simulink model "RadarSimulinkProjectRev004"  (R2024a)
settings: Solver=VariableStepAuto  StartTime=0.0  StopTime=0.012  RelTol=1e-3
values from neighbouring files (symbols this model uses):
  AngleTime = SweepTime/10    (= 10000)    [InitializationOfVariablesRev000.m]    (also in InitializationOfVariablesRev001.m; InitializationOfVariablesRev002.m = 2000; InitializationOfVariablesRev003.m = 20000; InitializationOfVariablesRev004.m = 2097152)
  ASR_LUT = Rsamp    [InitializationOfVariablesRev003.m]    (also in InitializationOfVariablesRev004.m = round((R*2*SystemFs)/c); InitializationOfVariablesRev005.m = round((R*2*SystemFs)/c))
  Btn_Debounce = 20000    [InitializationOfVariablesRev003.m]    (also in InitializationOfVariablesRev004.m; InitializationOfVariablesRev005.m)
  ChirpNc = 128    [InitializationOfVariablesRev004.m]    (also in InitializationOfVariablesRev005.m)
  ChirpSizeLength = length(FCW)    [InitializationOfVariablesRev004.m]    (also in InitializationOfVariablesRev005.m = 16384)
  FreqDeltaPeriod = 54    [InitializationOfVariablesRev003.m]    (also in InitializationOfVariablesRev004.m = 1)
  RXFFTLength = 4096    [InitializationOfVariablesRev003.m]    (also in InitializationOfVariablesRev004.m = 1024; InitializationOfVariablesRev005.m = 2048)
  SweepTime = 100000    [InitializationOfVariablesRev000.m]    (also in InitializationOfVariablesRev001.m; InitializationOfVariablesRev002.m = 20000; InitializationOfVariablesRev003.m = 200000; InitializationOfVariablesRev004.m = 23068672)
undefined symbols (not defined in the file or in its folder): SignalGenerationForAnalysis, Subsystem, xc7a200tfbg676
libraries: hdlBasic x323, hdlDSPIP x12, hdlUtilities x11, vmcUtilities x1
(part 3 of 3)

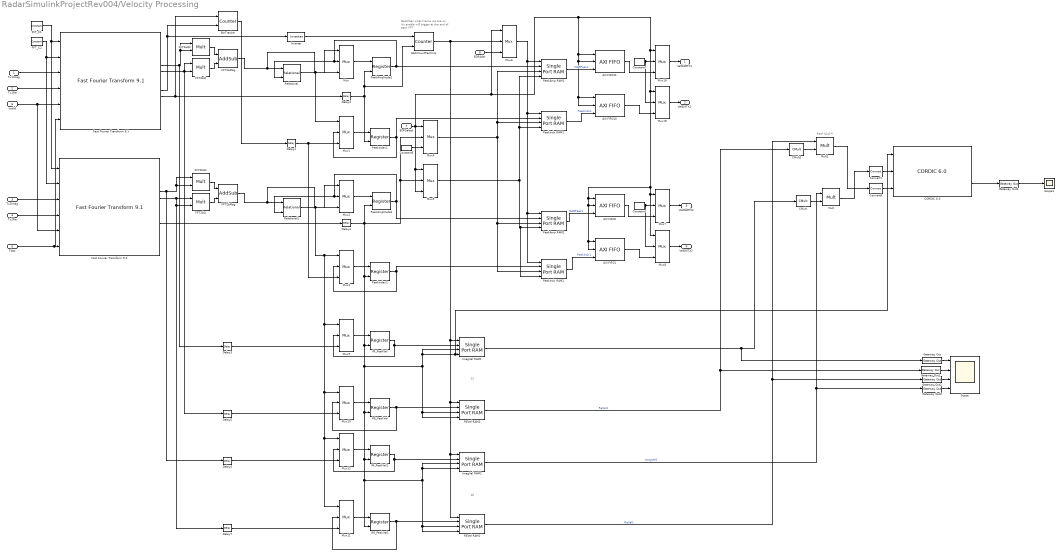
== system RadarSimulinkProjectRev004/Velocity Processing ==
  note: Real (z2z1*)
  note: Z1
  note: Describes what Frame we are on, it's enable will trigger at the end of each FFT
  note: Z2
  Tx1Imag : Inport
  Tx1Re : Inport  Port=2
  Tx2Imag : Inport  Port=3
  Tx2Re : Inport  Port=4
  Tlast : Inport  Port=5
  tvalid : Inport  Port=6
  EOFSelect : Inport  Port=7
  EOFAddr : Inport  Port=8
  AXI FIFO{1..2,10..11} (4 alike) : hdlBasic/AXI FIFO  input_depth_axis=1K  actual_fifo_depth_label=1026  enable_tdata=on  enable_tdest=off  enable_tstrb=off  enable_tready=on  enable_tid=off  enable_tuser=off  enable_tkeep=off  enable_tlast=off  has_aresetn=off  enable_data_counts_axis=off  fifo_implementation_type_axis=Common Clock Block RAM  trim_axipin_name=on  programmable_full_type_axis=Full  full_threshold_assert_value_axis=0  programmable_empty_type_axis=Empty  empty_threshold_assert_value_axis=1022  underflow_flag_axi=0  underflow_sense_axi=Active High  overflow_flag_axi=0  overflow_sense_axi=Active High  simulation_type=fast_sim  XmcBlockStatus=1  maskContainerNames=tabcontainer1  block_type=axi_fifo  block_config=sysgen:AXI_FIFO_config
  AddrCountPerChirp : hdlBasic/Counter  cnt_type=Count limited  cnt_to=10  operation=Up  start_count=0  cnt_by_val=1  arith_type=Unsigned  n_bits=7  bin_pt=0  load_pin=off  rst=on  en=on  explicit_period=Explicit  period=1/200e6  use_behavioral_HDL=off  implementation=Fabric  XmcBlockStatus=1  maskContainerNames=group1  block_type=counter  block_config=sysgen:Counter_config  block_width=531  block_height=1023
  BinTracker : hdlBasic/Counter  cnt_type=Count limited  cnt_to=ChirpNc-1  operation=Up  start_count=0  cnt_by_val=1  arith_type=Unsigned  n_bits=14  bin_pt=0  load_pin=off  rst=on  en=on  explicit_period=Explicit  period=1/200e6  use_behavioral_HDL=off  implementation=Fabric  XmcBlockStatus=1  maskContainerNames=group1  block_type=counter  block_config=sysgen:Counter_config  block_width=531  block_height=1023
  CMult : hdlBasic/CMult  const=-1  gui_display_data_type=Fixed-point  const_n_bits=16  const_bin_pt=14  float_type=Single  exp_bits=8  fraction_bits=24  en=off  latency=0  precision=Full  arith_type="Signed  (2's comp)"  n_bits=16  bin_pt=14  quantization=Truncate  overflow=Wrap  use_behavioral_HDL=off  mem_type=Distributed RAM  pipeline=off  XmcBlockStatus=1  maskContainerNames=tabcontainer1  block_type=cmult  block_config=sysgen:CMult_config
      settings: infoedit=[]
  CMult1 : hdlBasic/CMult  const=-1  gui_display_data_type=Fixed-point  const_n_bits=16  const_bin_pt=14  float_type=Single  exp_bits=8  fraction_bits=24  en=off  latency=0  precision=Full  arith_type="Signed  (2's comp)"  n_bits=16  bin_pt=14  quantization=Truncate  overflow=Wrap  use_behavioral_HDL=off  mem_type=Distributed RAM  pipeline=off  XmcBlockStatus=1  maskContainerNames=tabcontainer1  block_type=cmult  block_config=sysgen:CMult_config
      settings: infoedit=[]
  CORDIC 6.0 : hdlDSPIP/CORDIC 6.0   functional_selection=Arc_Tan  architectural_configuration=Parallel  pipelining_mode=Maximum  data_format=SignedFraction  phase_format=Radians  input_width=16  output_width=16  round_mode=Truncate  iterations=0  precision=0  compensation_scaling=No_Scale_Compensation  coarse_rotation=on  aclken=off  aresetn=off  out_tready=off  cartesian_has_tuser=off  cartesian_has_tlast=off  cartesian_tuser_width=1  phase_has_tuser=off  phase_has_tlast=off  phase_tuser_width=1  out_tlast_behv=Null  flow_control=NonBlocking  optimize_goal=Resources  trim_axipin_name=on  simulation_type=hybrid_sim  simulation_model=sysgen:cordic_v6_0  data_path_portlist={'s_axis_cartesian_tdata_imag', 's_axis_cartesian_tdata_real', 's_axis_phase_tdata_phase', 'm_axis_dout_tdata_imag', 'm_axis_dout_tdata_real', 'm_axis_dout_tdata_phase','m_axis_dout_tdata'}  ip_name=CORDIC  ip_version=6.0  dsptool_ready=true  ipcore_usecache=true  ipcore_useipmodelcache=true  wrapper_available=true  port_translation_map={ 'aclken' => 'en', 'aresetn' => 'rst' }  XmcBlockStatus=1  maskContainerNames=group15  block_type=cordic_v6_0  block_config=sysgen:rodinimport_config  block_width=800
  Constant1 : hdlBasic/Constant  const=0  gui_display_data_type=Fixed-point  arith_type=Signed (2's comp)  n_bits=16  bin_pt=15  preci_type=Single  exp_width=8  frac_width=24  explicit_period=on  period=1/200e6  XmcBlockStatus=1  maskContainerNames=tabcontainer1  block_type=constant  block_config=sysgen:Constant_config
  Constant5 : hdlBasic/Constant  const=0  gui_display_data_type=Boolean  arith_type=Boolean  n_bits=16  bin_pt=15  preci_type=Single  exp_width=8  frac_width=24  explicit_period=on  period=1/200e6  XmcBlockStatus=1  maskContainerNames=tabcontainer1  block_type=constant  block_config=sysgen:Constant_config
  Constant7 : hdlBasic/Constant  const=0  gui_display_data_type=Fixed-point  arith_type=Signed (2's comp)  n_bits=16  bin_pt=15  preci_type=Single  exp_width=8  frac_width=24  explicit_period=on  period=1/200e6  XmcBlockStatus=1  maskContainerNames=tabcontainer1  block_type=constant  block_config=sysgen:Constant_config
  Convert7 : hdlBasic/Convert  gui_display_data_type=Fixed-point  arith_type=Signed (2's comp)  n_bits=33  bin_pt=31  float_type=Single  exp_bits=8  fraction_bits=24  quantization=Truncate  overflow=Wrap  en=off  latency=0  pipeline=off  XmcBlockStatus=1  maskContainerNames=group2  block_type=convert  block_config=sysgen:Convert_config  block_width=595  block_height=885
  Convert8 : hdlBasic/Convert  gui_display_data_type=Fixed-point  arith_type=Signed (2's comp)  n_bits=33  bin_pt=31  float_type=Single  exp_bits=8  fraction_bits=24  quantization=Truncate  overflow=Wrap  en=off  latency=0  pipeline=off  XmcBlockStatus=1  maskContainerNames=group2  block_type=convert  block_config=sysgen:Convert_config  block_width=595  block_height=885
  Delay{1,3,5..7} (5 alike) : hdlBasic/Delay  rst=off  en=off  latency=3  reg_retiming=off  XmcBlockStatus=1  maskContainerNames=group1  block_type=delay  block_config=sysgen:Delay_config
  Delay2 : hdlBasic/Delay  rst=off  en=off  latency=1  reg_retiming=off  XmcBlockStatus=1  maskContainerNames=group1  block_type=delay  block_config=sysgen:Delay_config
  Delay4 : hdlBasic/Delay  rst=off  en=off  latency=1  reg_retiming=off  XmcBlockStatus=1  maskContainerNames=group1  block_type=delay  block_config=sysgen:Delay_config
  FFT2aI2 : hdlBasic/Mult  precision=Full  arith_type="Signed  (2's comp)"  n_bits=16  bin_pt=14  quantization=Truncate  overflow=Wrap  en=off  latency=3  opt_float=off  fp_mult_usage=No Usage  use_behavioral_HDL=off  opt=Speed  use_embedded=on  optimum_pipeline=off  pipeline=on  use_rpm=on  placement_style=Triangular  XmcBlockStatus=1  maskContainerNames=group1  block_type=mult  block_config=sysgen:Mult_config  block_width=598  block_height=876
  FFT2aMag : hdlBasic/AddSub  mode=Addition  use_carryin=off  use_carryout=off  en=off  latency=0  precision=Full  arith_type=Unsigned  n_bits=16  bin_pt=14  quantization=Truncate  overflow=Wrap  use_behavioral_HDL=off  hw_selection=Fabric  pipelined=off  XmcBlockStatus=1  maskContainerNames=tabcontainer1  block_type=addsub  block_config=sysgen:Addsub_config
  FFT2aQ2 : hdlBasic/Mult  precision=Full  arith_type="Signed  (2's comp)"  n_bits=16  bin_pt=14  quantization=Truncate  overflow=Wrap  en=off  latency=3  opt_float=off  fp_mult_usage=No Usage  use_behavioral_HDL=off  opt=Speed  use_embedded=on  optimum_pipeline=off  pipeline=on  use_rpm=on  placement_style=Triangular  XmcBlockStatus=1  maskContainerNames=group1  block_type=mult  block_config=sysgen:Mult_config  block_width=598  block_height=876
  FFT2bI2 : hdlBasic/Mult  precision=Full  arith_type="Signed  (2's comp)"  n_bits=16  bin_pt=14  quantization=Truncate  overflow=Wrap  en=off  latency=3  opt_float=off  fp_mult_usage=No Usage  use_behavioral_HDL=off  opt=Speed  use_embedded=on  optimum_pipeline=off  pipeline=on  use_rpm=on  placement_style=Triangular  XmcBlockStatus=1  maskContainerNames=group1  block_type=mult  block_config=sysgen:Mult_config  block_width=598  block_height=876
  FFT2bMag : hdlBasic/AddSub  mode=Addition  use_carryin=off  use_carryout=off  en=off  latency=0  precision=Full  arith_type=Unsigned  n_bits=16  bin_pt=14  quantization=Truncate  overflow=Wrap  use_behavioral_HDL=off  hw_selection=Fabric  pipelined=off  XmcBlockStatus=1  maskContainerNames=tabcontainer1  block_type=addsub  block_config=sysgen:Addsub_config
  FFT2bQ2 : hdlBasic/Mult  precision=Full  arith_type="Signed  (2's comp)"  n_bits=16  bin_pt=14  quantization=Truncate  overflow=Wrap  en=off  latency=3  opt_float=off  fp_mult_usage=No Usage  use_behavioral_HDL=off  opt=Speed  use_embedded=on  optimum_pipeline=off  pipeline=on  use_rpm=on  placement_style=Triangular  XmcBlockStatus=1  maskContainerNames=group1  block_type=mult  block_config=sysgen:Mult_config  block_width=598  block_height=876
  FFT_C1 : hdlBasic/Constant  const=1.0  gui_display_data_type=Fixed-point  arith_type=Unsigned  n_bits=1  bin_pt=0  preci_type=Single  exp_width=8  frac_width=24  explicit_period=on  period=1/200e6  XmcBlockStatus=1  maskContainerNames=tabcontainer1  block_type=constant  block_config=sysgen:Constant_config
  FFT_C2 : hdlBasic/Constant  const=1.0  gui_display_data_type=Boolean  arith_type=Boolean  n_bits=1  bin_pt=0  preci_type=Single  exp_width=8  frac_width=24  explicit_period=on  period=1/200e6  XmcBlockStatus=1  maskContainerNames=tabcontainer1  block_type=constant  block_config=sysgen:Constant_config
  Fast Fourier Transform 9.1 : hdlDSPIP/Fast Fourier Transform 9.1   transform_length=128  target_clock_frequency=250  target_data_throughput=50  implementation_options=pipelined_streaming_io  run_time_configurable_transform_length=off  enable_ssr=off  super_sample_rates=1  data_format=fixed_point  phase_factor_width=24  scaling_options=block_floating_point  rounding_modes=truncation  aclken=off  aresetn=off  output_ordering=natural_order  cyclic_prefix_insertion=off  throttle_scheme=realtime  xk_index=on  ovflo=off  trim_axipin_name=on  memory_options_data=block_ram  memory_options_phase_factors=block_ram  number_of_stages_using_block_ram_for_data_and_phase_factors=2  memory_options_reorder=block_ram  memory_options_hybrid=off  complex_mult_type=use_mults_resources  butterfly_type=use_xtremedsp_slices  simulation_type=hybrid_sim  simulation_model=sysgen:xfftv9_cmodel  data_path_portlist={ 's_axis_data_tdata', 'm_axis_data_tdata', 'm_axis_status_tdata', 'event_fft_overflow' }  channels=1  input_ordering=natural_order  input_width=16  ip_name=Fast Fourier Transform  ip_version=9.1  dsptool_ready=true  ipcore_usecache=true  ipcore_useipmodelcache=true  wrapper_available=true  port_translation_map={ 'aclken' => 'en', 'aresetn' => 'rst'}  XmcBlockStatus=1  maskContainerNames=tabcontainer1  block_type=xfft_v9_1  block_config=sysgen:rodinimport_config
  Fast Fourier Transform 9.2 : hdlDSPIP/Fast Fourier Transform 9.1   transform_length=128  target_clock_frequency=250  target_data_throughput=50  implementation_options=pipelined_streaming_io  run_time_configurable_transform_length=off  enable_ssr=off  super_sample_rates=1  data_format=fixed_point  phase_factor_width=24  scaling_options=block_floating_point  rounding_modes=truncation  aclken=off  aresetn=off  output_ordering=natural_order  cyclic_prefix_insertion=off  throttle_scheme=realtime  xk_index=on  ovflo=off  trim_axipin_name=on  memory_options_data=block_ram  memory_options_phase_factors=block_ram  number_of_stages_using_block_ram_for_data_and_phase_factors=2  memory_options_reorder=block_ram  memory_options_hybrid=off  complex_mult_type=use_mults_resources  butterfly_type=use_xtremedsp_slices  simulation_type=hybrid_sim  simulation_model=sysgen:xfftv9_cmodel  data_path_portlist={ 's_axis_data_tdata', 'm_axis_data_tdata', 'm_axis_status_tdata', 'event_fft_overflow' }  channels=1  input_ordering=natural_order  input_width=16  ip_name=Fast Fourier Transform  ip_version=9.1  dsptool_ready=true  ipcore_usecache=true  ipcore_useipmodelcache=true  wrapper_available=true  port_translation_map={ 'aclken' => 'en', 'aresetn' => 'rst'}  XmcBlockStatus=1  maskContainerNames=tabcontainer1  block_type=xfft_v9_1  block_config=sysgen:rodinimport_config
  Gateway Out{,1..4} (5 alike) : hdlBasic/Gateway Out  inherit_from_input=off  bool_to_boolean=off  hdl_port=on  rows=1  columns=1  UseAsDAC=off  DACChannel='1'  interface=None  automatic_assignment=on  address_offset=hex2dec('00')  intf_name=''  intf_description=''  timing_constraint=None  locs_specified=off  LOCs={}  io_standard={}  XmcBlockStatus=1  maskContainerNames=group4  block_type=gatewayout  block_config=sysgen:gateway_out_config  block_width_w=590  block_height_w=620  block_width=620  block_height=750
  IM_PeakVal : hdlBasic/Register  init=0  rst=on  en=off  XmcBlockStatus=1  maskContainerNames=tabcontainer1  block_type=register  block_config=sysgen:Register_config
  IM_PeakVal1 : hdlBasic/Register  init=0  rst=on  en=off  XmcBlockStatus=1  maskContainerNames=tabcontainer1  block_type=register  block_config=sysgen:Register_config
  ImagVal RAM1 : hdlBasic/Single Port RAM  depth=ChirpNc  initVector=0  distributed_mem=Block RAM  write_mode=Read After Write  rst=off  init_reg=0  en=on  optimize_latency=off  latency=1  optimize=Area  dbl_ovrd=off  simulation_type=fast_sim  XmcBlockStatus=1  maskContainerNames=tabcontainer1  block_type=spram  block_config=sysgen:SPRAM_config
  ImagVal RAM2 : hdlBasic/Single Port RAM  depth=ChirpNc  initVector=0  distributed_mem=Block RAM  write_mode=Read After Write  rst=off  init_reg=0  en=on  optimize_latency=off  latency=1  optimize=Area  dbl_ovrd=off  simulation_type=fast_sim  XmcBlockStatus=1  maskContainerNames=tabcontainer1  block_type=spram  block_config=sysgen:SPRAM_config
  Inverter : hdlBasic/Inverter  en=off  latency=0  XmcBlockStatus=1  maskContainerNames=group2  block_type=inv  block_config=sysgen:Inverter_config
  Mult : hdlBasic/Mult  precision=Full  arith_type="Signed  (2's comp)"  n_bits=16  bin_pt=14  quantization=Truncate  overflow=Wrap  en=off  latency=3  opt_float=off  fp_mult_usage=No Usage  use_behavioral_HDL=off  opt=Speed  use_embedded=on  optimum_pipeline=off  pipeline=on  use_rpm=on  placement_style=Triangular  XmcBlockStatus=1  maskContainerNames=group1  block_type=mult  block_config=sysgen:Mult_config  block_width=598  block_height=876
  Mult1 : hdlBasic/Mult  precision=Full  arith_type="Signed  (2's comp)"  n_bits=16  bin_pt=14  quantization=Truncate  overflow=Wrap  en=off  latency=3  opt_float=off  fp_mult_usage=No Usage  use_behavioral_HDL=off  opt=Speed  use_embedded=on  optimum_pipeline=off  pipeline=on  use_rpm=on  placement_style=Triangular  XmcBlockStatus=1  maskContainerNames=group1  block_type=mult  block_config=sysgen:Mult_config  block_width=598  block_height=876
  Mux{,1..12,18..19} (15 alike) : hdlBasic/Mux  inputs=2  en=off  latency=0  precision=Full  arith_type=Unsigned  n_bits=16  bin_pt=14  quantization=Truncate  overflow=Wrap  XmcBlockStatus=1  maskContainerNames=tabcontainer1  block_type=mux  block_config=sysgen:Mux_config
  PeakAmp RAM1 : hdlBasic/Single Port RAM  depth=ChirpNc  initVector=0  distributed_mem=Block RAM  write_mode=Read After Write  rst=off  init_reg=0  en=on  optimize_latency=off  latency=1  optimize=Area  dbl_ovrd=off  simulation_type=fast_sim  XmcBlockStatus=1  maskContainerNames=tabcontainer1  block_type=spram  block_config=sysgen:SPRAM_config
  PeakAmp RAM2 : hdlBasic/Single Port RAM  depth=ChirpNc  initVector=0  distributed_mem=Block RAM  write_mode=Read After Write  rst=off  init_reg=0  en=on  optimize_latency=off  latency=1  optimize=Area  dbl_ovrd=off  simulation_type=fast_sim  XmcBlockStatus=1  maskContainerNames=tabcontainer1  block_type=spram  block_config=sysgen:SPRAM_config
  PeakAmplitude1 : hdlBasic/Register  init=0  rst=on  en=off  XmcBlockStatus=1  maskContainerNames=tabcontainer1  block_type=register  block_config=sysgen:Register_config
  PeakAmplitude2 : hdlBasic/Register  init=0  rst=on  en=off  XmcBlockStatus=1  maskContainerNames=tabcontainer1  block_type=register  block_config=sysgen:Register_config
  PeakIndex1 : hdlBasic/Register  init=0  rst=on  en=off  XmcBlockStatus=1  maskContainerNames=tabcontainer1  block_type=register  block_config=sysgen:Register_config
  PeakIndex2 : hdlBasic/Register  init=0  rst=on  en=off  XmcBlockStatus=1  maskContainerNames=tabcontainer1  block_type=register  block_config=sysgen:Register_config
  PeakIndx RAM1 : hdlBasic/Single Port RAM  depth=ChirpNc  initVector=0  distributed_mem=Block RAM  write_mode=Read After Write  rst=off  init_reg=0  en=on  optimize_latency=off  latency=1  optimize=Area  dbl_ovrd=off  simulation_type=fast_sim  XmcBlockStatus=1  maskContainerNames=tabcontainer1  block_type=spram  block_config=sysgen:SPRAM_config
  PeakIndx RAM2 : hdlBasic/Single Port RAM  depth=ChirpNc  initVector=0  distributed_mem=Block RAM  write_mode=Read After Write  rst=off  init_reg=0  en=on  optimize_latency=off  latency=1  optimize=Area  dbl_ovrd=off  simulation_type=fast_sim  XmcBlockStatus=1  maskContainerNames=tabcontainer1  block_type=spram  block_config=sysgen:SPRAM_config
  REVal RAM1 : hdlBasic/Single Port RAM  depth=ChirpNc  initVector=0  distributed_mem=Block RAM  write_mode=Read After Write  rst=off  init_reg=0  en=on  optimize_latency=off  latency=1  optimize=Area  dbl_ovrd=off  simulation_type=fast_sim  XmcBlockStatus=1  maskContainerNames=tabcontainer1  block_type=spram  block_config=sysgen:SPRAM_config
  REVal RAM2 : hdlBasic/Single Port RAM  depth=ChirpNc  initVector=0  distributed_mem=Block RAM  write_mode=Read After Write  rst=off  init_reg=0  en=on  optimize_latency=off  latency=1  optimize=Area  dbl_ovrd=off  simulation_type=fast_sim  XmcBlockStatus=1  maskContainerNames=tabcontainer1  block_type=spram  block_config=sysgen:SPRAM_config
  RE_PeakVal : hdlBasic/Register  init=0  rst=on  en=off  XmcBlockStatus=1  maskContainerNames=tabcontainer1  block_type=register  block_config=sysgen:Register_config
  RE_PeakVal1 : hdlBasic/Register  init=0  rst=on  en=off  XmcBlockStatus=1  maskContainerNames=tabcontainer1  block_type=register  block_config=sysgen:Register_config
  Relational : hdlBasic/Relational  mode=a>b  op_type=Bool  en=off  latency=0  XmcBlockStatus=1  maskContainerNames=tabcontainer1  block_type=relational  block_config=sysgen:Relational_config
  Relational1 : hdlBasic/Relational  mode=a>b  op_type=Bool  en=off  latency=0  XmcBlockStatus=1  maskContainerNames=tabcontainer1  block_type=relational  block_config=sysgen:Relational_config
  Scope : Scope  NumInputPorts=4
  Scope1 : Scope
  VelMAGTX1 : Outport
  VelIDXTX1 : Outport  Port=2
  VelMAGTX2 : Outport  Port=3
  VelIDXTX2 : Outport  Port=4
  wires:
  FFT_C1/1 -> Fast Fourier Transform 9.2/1, Fast Fourier Transform 9.1/1
  Tx2Re/1 -> Fast Fourier Transform 9.2/4
  Tx2Imag/1 -> Fast Fourier Transform 9.2/3
  FFT_C2/1 -> Fast Fourier Transform 9.2/2, Fast Fourier Transform 9.1/2
  tvalid/1 -> Fast Fourier Transform 9.2/5, Fast Fourier Transform 9.1/5
  Tx1Re/1 -> Fast Fourier Transform 9.1/4
  Tx1Imag/1 -> Fast Fourier Transform 9.1/3
  Tlast/1 -> Fast Fourier Transform 9.1/6, Fast Fourier Transform 9.2/6
  Delay2/1 -> PeakAmplitude1/2, AddrCountPerChirp/2, PeakIndex1/2
  Fast Fourier Transform 9.1/5 -> Delay3/1, FFT2aQ2/2, FFT2aQ2/1
  Fast Fourier Transform 9.1/10 -> Delay2/1, BinTracker/1
  PeakAmplitude1/1 -> Relational/2, Mux/2, PeakAmp RAM1/2
  FFT2aI2/1 -> FFT2aMag/2
  FFT2aQ2/1 -> FFT2aMag/1
  Relational/1 -> Mux1/1, Mux/1
  Mux1/1 -> PeakIndex1/1
  Mux/1 -> PeakAmplitude1/1
  Fast Fourier Transform 9.1/6 -> Delay5/1, FFT2aI2/1, FFT2aI2/2
  FFT2aMag/1 -> Relational/1, Mux/3
  Delay1/1 -> Mux3/3, Mux1/3
  Fast Fourier Transform 9.1/9 -> Inverter/1, BinTracker/2
  Inverter/1 -> AddrCountPerChirp/1
  Mux2/1 -> PeakAmplitude2/1
  FFT2bMag/1 -> Relational1/1, Mux2/3
  Fast Fourier Transform 9.2/10 -> Delay4/1
  PeakIndex2/1 -> PeakIndx RAM2/2, Mux3/2
  Mux3/1 -> PeakIndex2/1
  BinTracker/1 -> Delay1/1
  FFT2bI2/1 -> FFT2bMag/2
  PeakAmplitude2/1 -> Relational1/2, Mux2/2, PeakAmp RAM2/2
  FFT2bQ2/1 -> FFT2bMag/1
  PeakIndex1/1 -> PeakIndx RAM1/2, Mux1/2
  Constant5/1 -> Mux4/3
  Mux4/1 -> PeakIndx RAM1/3, PeakAmp RAM1/3, PeakIndx RAM2/3, PeakAmp RAM2/3
  Mux5/1 -> PeakAmp RAM1/4, PeakIndx RAM1/4, PeakIndx RAM2/4, PeakAmp RAM2/4
  PeakAmp RAM1/1 -> AXI FIFO11/3  "MAGPeak1"
  Mux6/1 -> PeakIndx RAM2/1, PeakAmp RAM2/1, PeakIndx RAM1/1, PeakAmp RAM1/1
  PeakIndx RAM1/1 -> AXI FIFO10/3  "PeakIndx1"
  PeakAmp RAM2/1 -> AXI FIFO2/3  "MAGPeak1"
  PeakIndx RAM2/1 -> AXI FIFO1/3  "PeakIndx1"
  AXI FIFO11/2 -> Mux18/3
  AXI FIFO10/2 -> Mux19/3
  Mux18/1 -> VelMAGTX1/1
  Mux19/1 -> VelIDXTX1/1
  Constant7/1 -> Mux19/2, Mux18/2
  Mux8/1 -> VelIDXTX2/1
  AXI FIFO2/2 -> Mux7/3
  AXI FIFO1/2 -> Mux8/3
  Mux7/1 -> VelMAGTX2/1
  EOFSelect/1 -> Mux6/1, AXI FIFO10/2, AXI FIFO10/1, AXI FIFO11/2, AXI FIFO11/1, AXI FIFO1/2, AXI FIFO1/1, AXI FIFO2/2, AXI FIFO2/1, Mux7/1, Mux8/1, Mux19/1, Mux18/1, Mux5/3, Mux5/1, Mux4/1
  Constant1/1 -> Mux8/2, Mux7/2
  EOFAddr/1 -> Mux6/3
  Gateway Out3/1 -> Scope/4
  Gateway Out2/1 -> Scope/3
  Gateway Out1/1 -> Scope/2
  Gateway Out/1 -> Scope/1
  Convert7/1 -> CORDIC 6.0/2
  CORDIC 6.0/2 -> Gateway Out4/1
  Gateway Out4/1 -> Scope1/1
  Mult/1 -> Convert7/1
  Mult1/1 -> Convert8/1
  Convert8/1 -> CORDIC 6.0/3
  CMult/1 -> Mult/2
  ImagVal RAM1/1 -> Gateway Out/1, CMult/1
  Mux9/1 -> IM_PeakVal/1
  Delay5/1 -> Mux10/3
  IM_PeakVal/1 -> ImagVal RAM1/2, Mux9/2
  Delay3/1 -> Mux9/3
  RE_PeakVal/1 -> Mux10/2, REVal RAM2/2
  Mux10/1 -> RE_PeakVal/1
  Mux11/1 -> RE_PeakVal1/1
  Fast Fourier Transform 9.2/6 -> FFT2bI2/1, Delay7/1, FFT2bI2/2
  Delay4/1 -> PeakAmplitude2/2, Mux5/2, Mux4/2, IM_PeakVal/2, CORDIC 6.0/1, ImagVal RAM1/4, ImagVal RAM1/3, REVal RAM2/4, REVal RAM2/3, IM_PeakVal1/2, ImagVal RAM2/4, ImagVal RAM2/3, REVal RAM1/4, REVal RAM1/3, RE_PeakVal1/2, RE_PeakVal/2, PeakIndex2/2
  AddrCountPerChirp/1 -> REVal RAM1/1, ImagVal RAM2/1, REVal RAM2/1, ImagVal RAM1/1, Mux6/2
  Relational1/1 -> Mux12/1, Mux11/1, Mux10/1, Mux9/1, Mux3/1, Mux2/1
  RE_PeakVal1/1 -> Mux11/2, REVal RAM1/2
  IM_PeakVal1/1 -> ImagVal RAM2/2, Mux12/2
  Delay7/1 -> Mux11/3
  Fast Fourier Transform 9.2/5 -> Delay6/1, FFT2bQ2/1, FFT2bQ2/2
  Delay6/1 -> Mux12/3
  Mux12/1 -> IM_PeakVal1/1
  ImagVal RAM2/1 -> Gateway Out3/1, Mult/1  "ImagVal1"
  CMult1/1 -> Mult1/2
  REVal RAM1/1 -> Gateway Out2/1, Mult1/1  "ReVal1"
  REVal RAM2/1 -> Gateway Out1/1, CMult1/1  "ReVal1"

== matlab function RadarSimulinkProjectRev004/Enabled Subsystem/MATLAB Function ==
  data: dataIn input; rowIdx input; frameIdx input; writeEnable input
function write_RangeMAG1(dataIn, rowIdx, frameIdx, writeEnable)
%#codegen

% Tell the compiler this is an external Data Store variable
% (must match the name of your Data Store Memory block)
coder.extrinsic('RangeMAG1_store');  % optional for simulation-only
persistent initDone
if isempty(initDone)
    initDone = true;
end

% Declare data store variable
RangeMAG1_store = coder.wref('RangeMAG1_store');

% Only write when enabled
if writeEnable
    RangeMAG1_store(rowIdx+1, frameIdx+1) = dataIn;
end
